simulink model "mrefrobotarm_modified_previous_y_previous_u_previous_ref_pert_2"  (R2018b)
settings: Solver=FixedStepAuto  StartTime=0.0  StopTime=60  RelTol=1e-3  AbsTol=1e-6
undefined symbols (not defined in the file or in its folder): cc, options
libraries: neural x858, simulink x1
(part 30 of 32)

== system mrefrobotarm_modified_previous_y_previous_u_previous_ref_pert_2/m=0.01 sd=0.001/Layer 3/Delays 1 ==
  "p{3}" : Inport  PortDimensions=30
      mask Display: e = 0.06;c1 = [120 230 180]/255;c2 = ([120 230 180]+0)/(256+128);c3 = ([120 230 180]+128)/(256+128);patch([0 1 1 0],[0 0 1 1],c1);patch([0 1 1 1-e 1-e 0+e],[0 0 1 1-e 0+e 0+e],c2);patch([0 0 1 1-e 0+e 0+e],[0 1 1 1-e 1-e 0+e],c3);plot([0 1 1 0 0],[0 0 1 1 0]);
  mux : Mux  Inputs=1
      mask Display: e = 0.06;c1 = [120 150 230]/255;c2 = ([120 150 230]+0)/383;c3 = ([120 150 230]+128)/383;patch([0 1 1 0],[0 0 1 1],c1);patch([0 1 1 1-e 1-e 0+e],[0 0 1 1-e 0+e 0+e],c2);patch([0 0 1 1-e 0+e 0+e],[0 1 1 1-e 1-e 0+e],c3);plot([0 1 1 0 0],[0 0 1 1 0]);disp('Mux')
  "pd{3,2}" : Outport
      mask Display: e = 0.06;c1 = [120 230 180]/255;c2 = ([120 230 180]+0)/(256+128);c3 = ([120 230 180]+128)/(256+128);patch([0 1 1 0],[0 0 1 1],c1);patch([0 1 1 1-e 1-e 0+e],[0 0 1 1-e 0+e 0+e],c2);patch([0 0 1 1-e 0+e 0+e],[0 1 1 1-e 1-e 0+e],c3);plot([0 1 1 0 0],[0 0 1 1 0]);
  wires:
  "p{3}"/1 -> mux/1
  mux/1 -> "pd{3,2}"/1

== system mrefrobotarm_modified_previous_y_previous_u_previous_ref_pert_2/m=0.01 sd=0.001/Layer 3/LW{3,2} ==
  "ad{3,2}" : Inport  PortDimensions=30
      mask Display: e = 0.06;c1 = [120 230 180]/255;c2 = ([120 230 180]+0)/(256+128);c3 = ([120 230 180]+128)/(256+128);patch([0 1 1 0],[0 0 1 1],c1);patch([0 1 1 1-e 1-e 0+e],[0 0 1 1-e 0+e 0+e],c2);patch([0 0 1 1-e 0+e 0+e],[0 1 1 1-e 1-e 0+e],c3);plot([0 1 1 0 0],[0 0 1 1 0]);
  "IW{3,2}(1,:)'" : Constant  Value=[0.243283358953629402776641654781997203826904296875;0.0052243178148873060939738621755168423987925052642822265625;0.0264492508062884081054821905354401678778231143951416015625;0.2454647413544485401448724815054447390139102935791015625;-0.30345238295906995507067449580063112080097198486328125;-0.08772749743109610476299309311798424459993839263916015625;-0.300484076073690486996525805807323195040225982666015625;-0.25574179039630273724270637103472836315631866455078125;-0.4022085380966633483268424242851324379444122314453125;-0.32038735324012412863936560825095511972904205322265625;0.39682017437081473776316897783544845879077911376953125;-0.19002415108010850541830905058304779231548309326171875;0.1034079154633195385404320632005692459642887115478515625;-0.49654610538757726345693299663253128528594970703125;-0.252709011184159615392985642756684683263301849365234375;0.051813445988101620998111940252783824689686298370361328125;-0.119411317170181663360750690117129124701023101806640625;-0.238083190801845312467577286952291615307331085205078125;0.0603028351061200285077035232461639679968357086181640625;0.334975652187224304245916073341504670679569244384765625;-0.40385752692782972417262499220669269561767578125;0.26298542443057371098547037036041729152202606201171875;-0.379084529953288396075805621876497752964496612548828125;-0.330978605194054809057746524558751843869686126708984375;-0.289042778322861571016488824170664884150028228759765625;0.253230096744817612108846560659003444015979766845703125;-0.155565791924000607071576496309717185795307159423828125;0.159285938319768283211175230462686158716678619384765625;-0.28458279469647440595991838563350029289722442626953125;-0.6006058809980039381315464197541587054729461669921875]
      mask Display: e = 0.06;c1 = [120 150 230]/255;c2 = ([120 150 230]+0)/383;c3 = ([120 150 230]+128)/383;patch([0 1 1 0],[0 0 1 1],c1);patch([0 1 1 1-e 1-e 0+e],[0 0 1 1-e 0+e 0+e],c2);patch([0 0 1 1-e 0+e 0+e],[0 1 1 1-e 1-e 0+e],c3);plot([0 1 1 0 0],[0 0 1 1 0]);disp('weights');
  Mux : Mux  Inputs=1
      mask Display: e = 0.06;c1 = [120 150 230]/255;c2 = ([120 150 230]+0)/383;c3 = ([120 150 230]+128)/383;patch([0 1 1 0],[0 0 1 1],c1);patch([0 1 1 1-e 1-e 0+e],[0 0 1 1-e 0+e 0+e],c2);patch([0 0 1 1-e 0+e 0+e],[0 1 1 1-e 1-e 0+e],c3);plot([0 1 1 0 0],[0 0 1 1 0]);disp('Mux');
  dotprod1 : neural/Weight Functions/dotprod
  "lz{3,2}" : Outport
      mask Display: e = 0.06;c1 = [120 230 180]/255;c2 = ([120 230 180]+0)/(256+128);c3 = ([120 230 180]+128)/(256+128);patch([0 1 1 0],[0 0 1 1],c1);patch([0 1 1 1-e 1-e 0+e],[0 0 1 1-e 0+e 0+e],c2);patch([0 0 1 1-e 0+e 0+e],[0 1 1 1-e 1-e 0+e],c3);plot([0 1 1 0 0],[0 0 1 1 0]);
  wires:
  "IW{3,2}(1,:)'"/1 -> dotprod1/1
  "ad{3,2}"/1 -> dotprod1/2
  dotprod1/1 -> Mux/1
  Mux/1 -> "lz{3,2}"/1

== system mrefrobotarm_modified_previous_y_previous_u_previous_ref_pert_2/m=0.1 sd=0.001/Layer 1/Delays 1 ==
  "p{1}" : Inport  PortDimensions=10
      mask Display: e = 0.06;c1 = [120 230 180]/255;c2 = ([120 230 180]+0)/(256+128);c3 = ([120 230 180]+128)/(256+128);patch([0 1 1 0],[0 0 1 1],c1);patch([0 1 1 1-e 1-e 0+e],[0 0 1 1-e 0+e 0+e],c2);patch([0 0 1 1-e 0+e 0+e],[0 1 1 1-e 1-e 0+e],c3);plot([0 1 1 0 0],[0 0 1 1 0]);
  mux : Mux  Inputs=1
      mask Display: e = 0.06;c1 = [120 150 230]/255;c2 = ([120 150 230]+0)/383;c3 = ([120 150 230]+128)/383;patch([0 1 1 0],[0 0 1 1],c1);patch([0 1 1 1-e 1-e 0+e],[0 0 1 1-e 0+e 0+e],c2);patch([0 0 1 1-e 0+e 0+e],[0 1 1 1-e 1-e 0+e],c3);plot([0 1 1 0 0],[0 0 1 1 0]);disp('Mux')
  "pd{1,1}" : Outport
      mask Display: e = 0.06;c1 = [120 230 180]/255;c2 = ([120 230 180]+0)/(256+128);c3 = ([120 230 180]+128)/(256+128);patch([0 1 1 0],[0 0 1 1],c1);patch([0 1 1 1-e 1-e 0+e],[0 0 1 1-e 0+e 0+e],c2);patch([0 0 1 1-e 0+e 0+e],[0 1 1 1-e 1-e 0+e],c3);plot([0 1 1 0 0],[0 0 1 1 0]);
  wires:
  "p{1}"/1 -> mux/1
  mux/1 -> "pd{1,1}"/1

== system mrefrobotarm_modified_previous_y_previous_u_previous_ref_pert_2/m=0.1 sd=0.001/Layer 1/IW{1,1} ==
  "pd{1,1}" : Inport  PortDimensions=10
      mask Display: e = 0.06;c1 = [120 230 180]/255;c2 = ([120 230 180]+0)/(256+128);c3 = ([120 230 180]+128)/(256+128);patch([0 1 1 0],[0 0 1 1],c1);patch([0 1 1 1-e 1-e 0+e],[0 0 1 1-e 0+e 0+e],c2);patch([0 0 1 1-e 0+e 0+e],[0 1 1 1-e 1-e 0+e],c3);plot([0 1 1 0 0],[0 0 1 1 0]);
  "IW{1,1}(1,:)'" : Constant  Value=[0.97150289702667269597924359914031811058521270751953125;0.617885535943719421680953018949367105960845947265625;0.1752264140459464381027743229424231685698032379150390625;-0.0470176874894272234239878116568434052169322967529296875;0.75753700203231832954742230867850594222545623779296875;-0.6427595381168291766016409383155405521392822265625;0.53012825773271554652410486596636474132537841796875;0.6688038187694134162342152194469235837459564208984375;-1.51573934873066917816686327569186687469482421875;-1.8233994053194997331246440808172337710857391357421875]
      mask Display: e = 0.06;c1 = [120 150 230]/255;c2 = ([120 150 230]+0)/383;c3 = ([120 150 230]+128)/383;patch([0 1 1 0],[0 0 1 1],c1);patch([0 1 1 1-e 1-e 0+e],[0 0 1 1-e 0+e 0+e],c2);patch([0 0 1 1-e 0+e 0+e],[0 1 1 1-e 1-e 0+e],c3);plot([0 1 1 0 0],[0 0 1 1 0]);disp('Weights');
  "IW{1,1}(10,:)'" : Constant  Value=[0.489643008794402867511763588481699116528034210205078125;0.249588248674551038686075798977981321513652801513671875;0.4146828443458738799876073244377039372920989990234375;-0.44031407922737153537440235595568083226680755615234375;0.353625460658760715215720438209245912730693817138671875;0.926682652630255621062360660289414227008819580078125;-1.382443840359943720841329195536673069000244140625;-0.280540021092768598887090547577827237546443939208984375;2.600590207035732515095105554792098701000213623046875;0.87696388944716263669221234522410668432712554931640625]
      mask Display: e = 0.06;c1 = [120 150 230]/255;c2 = ([120 150 230]+0)/383;c3 = ([120 150 230]+128)/383;patch([0 1 1 0],[0 0 1 1],c1);patch([0 1 1 1-e 1-e 0+e],[0 0 1 1-e 0+e 0+e],c2);patch([0 0 1 1-e 0+e 0+e],[0 1 1 1-e 1-e 0+e],c3);plot([0 1 1 0 0],[0 0 1 1 0]);disp('Weights');
  "IW{1,1}(11,:)'" : Constant  Value=[-0.4287325006343249977902587488642893731594085693359375;0.2177436358527625459569065924370079301297664642333984375;0.0194862340827772033413634034104688907973468303680419921875;0.384060270608029774574987413870985619723796844482421875;0.8253590670554189490104590731789357960224151611328125;-2.082055111283486414919252638355828821659088134765625;1.23818472207362884063286401215009391307830810546875;0.2379638156625711598035621818780782632529735565185546875;-1.222522228966350876788737878086976706981658935546875;-0.06619512355622218791051381003853748552501201629638671875]
      mask Display: e = 0.06;c1 = [120 150 230]/255;c2 = ([120 150 230]+0)/383;c3 = ([120 150 230]+128)/383;patch([0 1 1 0],[0 0 1 1],c1);patch([0 1 1 1-e 1-e 0+e],[0 0 1 1-e 0+e 0+e],c2);patch([0 0 1 1-e 0+e 0+e],[0 1 1 1-e 1-e 0+e],c3);plot([0 1 1 0 0],[0 0 1 1 0]);disp('Weights');
  "IW{1,1}(12,:)'" : Constant  Value=[-1.2529262660683941899009141707210801541805267333984375;0.2109962353451392547132314803093322552740573883056640625;-0.07807793152172838591074111036505200900137424468994140625;0.06666872948784439978364702028557076118886470794677734375;1.981120844897162669440149329602718353271484375;-2.146903429308871569247685329173691570758819580078125;-0.26792451404853123708704742966801859438419342041015625;0.1142981625892685315637464782412280328571796417236328125;0.4915680538073254890463203992112539708614349365234375;1.042045568544349265494020073674619197845458984375]
      mask Display: e = 0.06;c1 = [120 150 230]/255;c2 = ([120 150 230]+0)/383;c3 = ([120 150 230]+128)/383;patch([0 1 1 0],[0 0 1 1],c1);patch([0 1 1 1-e 1-e 0+e],[0 0 1 1-e 0+e 0+e],c2);patch([0 0 1 1-e 0+e 0+e],[0 1 1 1-e 1-e 0+e],c3);plot([0 1 1 0 0],[0 0 1 1 0]);disp('Weights');
  "IW{1,1}(13,:)'" : Constant  Value=[-1.4694188756818398200465480840648524463176727294921875;0.6336793886650562424023291896446608006954193115234375;2.01225819370897429649858167977072298526763916015625;-0.050672278846553175934985802086885087192058563232421875;-3.23486632336392521125389976077713072299957275390625;2.224412737952894847381912768469192087650299072265625;2.065804235025697987992998605477623641490936279296875;-0.1310957483963151037897887363214977085590362548828125;-0.9522457855727191056161018423154018819332122802734375;-0.1780689484287442947429980222295853309333324432373046875]
      mask Display: e = 0.06;c1 = [120 150 230]/255;c2 = ([120 150 230]+0)/383;c3 = ([120 150 230]+128)/383;patch([0 1 1 0],[0 0 1 1],c1);patch([0 1 1 1-e 1-e 0+e],[0 0 1 1-e 0+e 0+e],c2);patch([0 0 1 1-e 0+e 0+e],[0 1 1 1-e 1-e 0+e],c3);plot([0 1 1 0 0],[0 0 1 1 0]);disp('Weights');
  "IW{1,1}(14,:)'" : Constant  Value=[1.8681607584848112235675898773479275405406951904296875;-1.5591874304554658170474112921510823071002960205078125;0.42450993697366146140126375030376948416233062744140625;-0.1220891736443905362108353074290789663791656494140625;0.763373075356110764033701343578286468982696533203125;-0.2270206585839918134173132102660019882023334503173828125;0.394047816935292838369520040942006744444370269775390625;0.64566378395872436879443512225407175719738006591796875;-0.22964258051511354796758723750826902687549591064453125;0.0630050111280484326226059010878088884055614471435546875]
      mask Display: e = 0.06;c1 = [120 150 230]/255;c2 = ([120 150 230]+0)/383;c3 = ([120 150 230]+128)/383;patch([0 1 1 0],[0 0 1 1],c1);patch([0 1 1 1-e 1-e 0+e],[0 0 1 1-e 0+e 0+e],c2);patch([0 0 1 1-e 0+e 0+e],[0 1 1 1-e 1-e 0+e],c3);plot([0 1 1 0 0],[0 0 1 1 0]);disp('Weights');
  "IW{1,1}(15,:)'" : Constant  Value=[-0.638387118902711048207265775999985635280609130859375;0.93259969282063870377186276527936570346355438232421875;-0.263201104520440820611071330858976580202579498291015625;-0.004599030717388432991377111846986736054532229900360107421875;1.472942132684331273395628159050829708576202392578125;-1.7999757214139944228037393259000964462757110595703125;0.66490212963451345018484062165953218936920166015625;-0.38142345551628842326152835084940306842327117919921875;-0.406565578149011452868677451988332904875278472900390625;-1.131003307321973405663584344438277184963226318359375]
      mask Display: e = 0.06;c1 = [120 150 230]/255;c2 = ([120 150 230]+0)/383;c3 = ([120 150 230]+128)/383;patch([0 1 1 0],[0 0 1 1],c1);patch([0 1 1 1-e 1-e 0+e],[0 0 1 1-e 0+e 0+e],c2);patch([0 0 1 1-e 0+e 0+e],[0 1 1 1-e 1-e 0+e],c3);plot([0 1 1 0 0],[0 0 1 1 0]);disp('Weights');
  "IW{1,1}(16,:)'" : Constant  Value=[-0.43428661364521559118401228261063806712627410888671875;1.007980197023808255352150808903388679027557373046875;-1.1368150682438351584124802684527821838855743408203125;0.046007823780444483119378418223277549259364604949951171875;0.369116877955644240305588255068869329988956451416015625;0.49535162439032187631227088786545209586620330810546875;-0.65503047820462800832075345169869251549243927001953125;0.84142974346925425432885958798578940331935882568359375;0.1335618919760182266021075747630675323307514190673828125;0.200164880680326950912473193966434337198734283447265625]
      mask Display: e = 0.06;c1 = [120 150 230]/255;c2 = ([120 150 230]+0)/383;c3 = ([120 150 230]+128)/383;patch([0 1 1 0],[0 0 1 1],c1);patch([0 1 1 1-e 1-e 0+e],[0 0 1 1-e 0+e 0+e],c2);patch([0 0 1 1-e 0+e 0+e],[0 1 1 1-e 1-e 0+e],c3);plot([0 1 1 0 0],[0 0 1 1 0]);disp('Weights');
  "IW{1,1}(17,:)'" : Constant  Value=[0.107552759922356966360013075245660729706287384033203125;-1.346270777388516304284848956740461289882659912109375;0.184320209842593396576404529696446843445301055908203125;-0.0895953581737940485396620715619064867496490478515625;0.981520970911235135503147830604575574398040771484375;1.02736081963616943113493107375688850879669189453125;-1.1863162004389049553054746866109780967235565185546875;0.283045855992447581428450575913302600383758544921875;-1.392742600295459709514034329913556575775146484375;0.1495563049644798858661687290805275551974773406982421875]
      mask Display: e = 0.06;c1 = [120 150 230]/255;c2 = ([120 150 230]+0)/383;c3 = ([120 150 230]+128)/383;patch([0 1 1 0],[0 0 1 1],c1);patch([0 1 1 1-e 1-e 0+e],[0 0 1 1-e 0+e 0+e],c2);patch([0 0 1 1-e 0+e 0+e],[0 1 1 1-e 1-e 0+e],c3);plot([0 1 1 0 0],[0 0 1 1 0]);disp('Weights');
  "IW{1,1}(18,:)'" : Constant  Value=[0.60421323192831499770960590467439033091068267822265625;0.863981081042938026115507454960606992244720458984375;-2.164800667863084893127734176232479512691497802734375;-0.07698153501303210688444522702411632053554058074951171875;-2.2141952501059449787135235965251922607421875;0.48418268786651286195166221659746952354907989501953125;0.1804086706541263851466538881140877492725849151611328125;-0.483357613735531099763420570525340735912322998046875;-2.250245781538189770998314997996203601360321044921875;-1.889499368656487376938457600772380828857421875]
      mask Display: e = 0.06;c1 = [120 150 230]/255;c2 = ([120 150 230]+0)/383;c3 = ([120 150 230]+128)/383;patch([0 1 1 0],[0 0 1 1],c1);patch([0 1 1 1-e 1-e 0+e],[0 0 1 1-e 0+e 0+e],c2);patch([0 0 1 1-e 0+e 0+e],[0 1 1 1-e 1-e 0+e],c3);plot([0 1 1 0 0],[0 0 1 1 0]);disp('Weights');
  "IW{1,1}(19,:)'" : Constant  Value=[-0.310316878774572646459972702359664253890514373779296875;-1.0780002166131661400783059434616006910800933837890625;0.97905383674770185553626333785359747707843780517578125;0.25263709689869118246718926457106135785579681396484375;0.198392588265190017438044378650374710559844970703125;1.958092704212322399115464577334932982921600341796875;-0.57605587336904939821380366993253119289875030517578125;-1.2966037305212319008518306873156689107418060302734375;1.1480352853282782543686835197149775922298431396484375;0.48066285180312073865849242793046869337558746337890625]
      mask Display: e = 0.06;c1 = [120 150 230]/255;c2 = ([120 150 230]+0)/383;c3 = ([120 150 230]+128)/383;patch([0 1 1 0],[0 0 1 1],c1);patch([0 1 1 1-e 1-e 0+e],[0 0 1 1-e 0+e 0+e],c2);patch([0 0 1 1-e 0+e 0+e],[0 1 1 1-e 1-e 0+e],c3);plot([0 1 1 0 0],[0 0 1 1 0]);disp('Weights');
  "IW{1,1}(2,:)'" : Constant  Value=[0.3387257184963281542167123916442506015300750732421875;-0.1797003643190983879218691754431347362697124481201171875;0.356085463904586119188167003812850452959537506103515625;-0.042189007117119099732338582953161676414310932159423828125;-1.649270794860369537815358853549696505069732666015625;1.464964797139139296433540948783047497272491455078125;-0.7069449258673403679864577497937716543674468994140625;0.61437488507698201356532763384166173636913299560546875;-0.2265416857285133256372233745423727668821811676025390625;0.376347036314308047710852633827016688883304595947265625]
      mask Display: e = 0.06;c1 = [120 150 230]/255;c2 = ([120 150 230]+0)/383;c3 = ([120 150 230]+128)/383;patch([0 1 1 0],[0 0 1 1],c1);patch([0 1 1 1-e 1-e 0+e],[0 0 1 1-e 0+e 0+e],c2);patch([0 0 1 1-e 0+e 0+e],[0 1 1 1-e 1-e 0+e],c3);plot([0 1 1 0 0],[0 0 1 1 0]);disp('Weights');
  "IW{1,1}(20,:)'" : Constant  Value=[-0.490140303142504396571865754594909958541393280029296875;0.79804833937093355711311915001715533435344696044921875;-1.2831688138474799387722669052891433238983154296875;0.291284969844939178873488572207861579954624176025390625;0.876417228536505721336880014860071241855621337890625;-1.7385563549437661468033411438227631151676177978515625;-0.50686148598950564458931467015645466744899749755859375;-0.28939862193536092238588253167108632624149322509765625;-1.2296078733237567615077523441868834197521209716796875;-1.57640760470990759500864442088641226291656494140625]
      mask Display: e = 0.06;c1 = [120 150 230]/255;c2 = ([120 150 230]+0)/383;c3 = ([120 150 230]+128)/383;patch([0 1 1 0],[0 0 1 1],c1);patch([0 1 1 1-e 1-e 0+e],[0 0 1 1-e 0+e 0+e],c2);patch([0 0 1 1-e 0+e 0+e],[0 1 1 1-e 1-e 0+e],c3);plot([0 1 1 0 0],[0 0 1 1 0]);disp('Weights');
  "IW{1,1}(21,:)'" : Constant  Value=[-0.8448419884512754496341813137405551970005035400390625;0.110704272323804142619252388612949289381504058837890625;0.6221730601826127582398839876987040042877197265625;-0.0094678207165062276684519559921682230196893215179443359375;-1.008898321112665197318847276619635522365570068359375;2.37691406571895935684324285830371081829071044921875;-0.98396704720915695308036674759932793676853179931640625;-0.301532716218349261527720273079467006027698516845703125;0.401508735767118707382650200088392011821269989013671875;0.48074242408417700023193219749373383820056915283203125]
      mask Display: e = 0.06;c1 = [120 150 230]/255;c2 = ([120 150 230]+0)/383;c3 = ([120 150 230]+128)/383;patch([0 1 1 0],[0 0 1 1],c1);patch([0 1 1 1-e 1-e 0+e],[0 0 1 1-e 0+e 0+e],c2);patch([0 0 1 1-e 0+e 0+e],[0 1 1 1-e 1-e 0+e],c3);plot([0 1 1 0 0],[0 0 1 1 0]);disp('Weights');
  "IW{1,1}(22,:)'" : Constant  Value=[-0.54005738902516398081132820152561180293560028076171875;1.6497089693146007594037882881821133196353912353515625;0.68022190254479852900004743787576444447040557861328125;-0.11952988714669064707063483865567832253873348236083984375;-2.191214874887081887067097341059707105159759521484375;0.823576955060695947707927189185284078121185302734375;2.546953080893350485069959177053533494472503662109375;-0.1184862413534755187782820939901284873485565185546875;-1.80301440869707452208103859447874128818511962890625;-0.5395918499269087842407088828622363507747650146484375]
      mask Display: e = 0.06;c1 = [120 150 230]/255;c2 = ([120 150 230]+0)/383;c3 = ([120 150 230]+128)/383;patch([0 1 1 0],[0 0 1 1],c1);patch([0 1 1 1-e 1-e 0+e],[0 0 1 1-e 0+e 0+e],c2);patch([0 0 1 1-e 0+e 0+e],[0 1 1 1-e 1-e 0+e],c3);plot([0 1 1 0 0],[0 0 1 1 0]);disp('Weights');
  "IW{1,1}(23,:)'" : Constant  Value=[0.1111125952273283867821618287052842788398265838623046875;-0.125837860955586411382256528668222017586231231689453125;-1.0573139259908701514945050803362391889095306396484375;0.0199283896174118069222203075696597807109355926513671875;0.315679639236594311579864324812660925090312957763671875;0.42717506618387834915751000153250060975551605224609375;-0.25276948903202633989195646790903992950916290283203125;0.37217397859028211737353331045596860349178314208984375;-0.047986027660040307674105264368336065672338008880615234375;-0.71436988024424419307933931122533977031707763671875]
      mask Display: e = 0.06;c1 = [120 150 230]/255;c2 = ([120 150 230]+0)/383;c3 = ([120 150 230]+128)/383;patch([0 1 1 0],[0 0 1 1],c1);patch([0 1 1 1-e 1-e 0+e],[0 0 1 1-e 0+e 0+e],c2);patch([0 0 1 1-e 0+e 0+e],[0 1 1 1-e 1-e 0+e],c3);plot([0 1 1 0 0],[0 0 1 1 0]);disp('Weights');
  "IW{1,1}(24,:)'" : Constant  Value=[0.6031876739999459946517390562803484499454498291015625;-1.36680629289936206305355881340801715850830078125;0.439752228564215530415282273679622448980808258056640625;0.313991143349557189079490626681945286691188812255859375;-0.5705459948731419483891613708692602813243865966796875;1.03530481535340346255225085769779980182647705078125;-0.59872468406984113986624151948490180075168609619140625;-0.1399879051014731590196760180333512835204601287841796875;0.190202809094372649045823209235095418989658355712890625;0.0005722435480554452676138499356284228269942104816436767578125]
      mask Display: e = 0.06;c1 = [120 150 230]/255;c2 = ([120 150 230]+0)/383;c3 = ([120 150 230]+128)/383;patch([0 1 1 0],[0 0 1 1],c1);patch([0 1 1 1-e 1-e 0+e],[0 0 1 1-e 0+e 0+e],c2);patch([0 0 1 1-e 0+e 0+e],[0 1 1 1-e 1-e 0+e],c3);plot([0 1 1 0 0],[0 0 1 1 0]);disp('Weights');
  "IW{1,1}(25,:)'" : Constant  Value=[-0.471166329686002638421626897979876957833766937255859375;0.019517284199158567437049072168520069681107997894287109375;-0.51375562108899142099716073062154464423656463623046875;-0.99099158086243332999032418229035101830959320068359375;-0.280529395720106877742949791354476474225521087646484375;0.408813229901232200180771769737475551664829254150390625;-1.4569675807901523167942059444612823426723480224609375;0.1597914239924210499932399898170842789113521575927734375;-1.151683674628356524038963470957241952419281005859375;-1.1155745139129293885815741305123083293437957763671875]
      mask Display: e = 0.06;c1 = [120 150 230]/255;c2 = ([120 150 230]+0)/383;c3 = ([120 150 230]+128)/383;patch([0 1 1 0],[0 0 1 1],c1);patch([0 1 1 1-e 1-e 0+e],[0 0 1 1-e 0+e 0+e],c2);patch([0 0 1 1-e 0+e 0+e],[0 1 1 1-e 1-e 0+e],c3);plot([0 1 1 0 0],[0 0 1 1 0]);disp('Weights');
  "IW{1,1}(26,:)'" : Constant  Value=[0.51788957071500363316118864531745202839374542236328125;-0.90550825047783722876459933104342781007289886474609375;0.874554192761201054651110098347999155521392822265625;0.05490630649626752901593107480948674492537975311279296875;-0.2376871617598398100934531385064474307000637054443359375;-1.4259068300949875318650583722046576440334320068359375;1.56037911854196753580481527023948729038238525390625;-0.5633426023816168193292241994640789926052093505859375;-0.3249990459048144320064466228359378874301910400390625;-0.1924690193035773211338579358198330737650394439697265625]
      mask Display: e = 0.06;c1 = [120 150 230]/255;c2 = ([120 150 230]+0)/383;c3 = ([120 150 230]+128)/383;patch([0 1 1 0],[0 0 1 1],c1);patch([0 1 1 1-e 1-e 0+e],[0 0 1 1-e 0+e 0+e],c2);patch([0 0 1 1-e 0+e 0+e],[0 1 1 1-e 1-e 0+e],c3);plot([0 1 1 0 0],[0 0 1 1 0]);disp('Weights');
  "IW{1,1}(27,:)'" : Constant  Value=[0.4086370536036636469390259662759490311145782470703125;-0.2007808125360639184275868274198728613555431365966796875;0.60343773748294415870674356483505107462406158447265625;1.070394363751332900136503667454235255718231201171875;2.2073601470784325329077546484768390655517578125;0.25483112077533653927474688316578976809978485107421875;-0.33905692912207296974003156719845719635486602783203125;-0.7065582091683511034574394216178916394710540771484375;-0.60042970740870671431110849880496971309185028076171875;-0.1279585049280285991013528246185160242021083831787109375]
      mask Display: e = 0.06;c1 = [120 150 230]/255;c2 = ([120 150 230]+0)/383;c3 = ([120 150 230]+128)/383;patch([0 1 1 0],[0 0 1 1],c1);patch([0 1 1 1-e 1-e 0+e],[0 0 1 1-e 0+e 0+e],c2);patch([0 0 1 1-e 0+e 0+e],[0 1 1 1-e 1-e 0+e],c3);plot([0 1 1 0 0],[0 0 1 1 0]);disp('Weights');
  "IW{1,1}(28,:)'" : Constant  Value=[-0.17889977814008284351388056165887974202632904052734375;-0.72737896249138522808408424680237658321857452392578125;0.876562342050114740032995541696436703205108642578125;0.06250436501011306933417444042788702063262462615966796875;0.98605104672372723140227890326059423387050628662109375;-0.0177154137537540203040098418796333135105669498443603515625;-1.1565789570964295496224849557620473206043243408203125;0.05094103404277350310991323567577637732028961181640625;0.53028155866240200833061635421472601592540740966796875;-0.637525850452747899765881811617873609066009521484375]
      mask Display: e = 0.06;c1 = [120 150 230]/255;c2 = ([120 150 230]+0)/383;c3 = ([120 150 230]+128)/383;patch([0 1 1 0],[0 0 1 1],c1);patch([0 1 1 1-e 1-e 0+e],[0 0 1 1-e 0+e 0+e],c2);patch([0 0 1 1-e 0+e 0+e],[0 1 1 1-e 1-e 0+e],c3);plot([0 1 1 0 0],[0 0 1 1 0]);disp('Weights');
  "IW{1,1}(29,:)'" : Constant  Value=[0.183816634740196216402097206810140050947666168212890625;-0.605890372960407486147005329257808625698089599609375;-0.52787986615784898702941063675098121166229248046875;0.3209207542221850228969515228527598083019256591796875;0.392028568404616972742360303527675569057464599609375;-0.71187172137459153731242622598074376583099365234375;0.1788547241704122325867132303756079636514186859130859375;0.89792898555716738062670856379554606974124908447265625;-0.80277707368138362387099959960323758423328399658203125;0.8280432752455038070138471084646880626678466796875]
      mask Display: e = 0.06;c1 = [120 150 230]/255;c2 = ([120 150 230]+0)/383;c3 = ([120 150 230]+128)/383;patch([0 1 1 0],[0 0 1 1],c1);patch([0 1 1 1-e 1-e 0+e],[0 0 1 1-e 0+e 0+e],c2);patch([0 0 1 1-e 0+e 0+e],[0 1 1 1-e 1-e 0+e],c3);plot([0 1 1 0 0],[0 0 1 1 0]);disp('Weights');
  "IW{1,1}(3,:)'" : Constant  Value=[-0.62632140158312987754385403604828752577304840087890625;-0.52645332897737973087970431151916272938251495361328125;0.422629068709391930713792362439562566578388214111328125;0.16303550788070542143515240240958519279956817626953125;1.162694599040965837133398963487707078456878662109375;-0.1394240777189013069659040411352179944515228271484375;0.02236044267614045732983640846214257180690765380859375;0.309760520161516395010181668112636543810367584228515625;-1.2335632156852314178507867836742661893367767333984375;-0.66691887772808045031780466160853393375873565673828125]
      mask Display: e = 0.06;c1 = [120 150 230]/255;c2 = ([120 150 230]+0)/383;c3 = ([120 150 230]+128)/383;patch([0 1 1 0],[0 0 1 1],c1);patch([0 1 1 1-e 1-e 0+e],[0 0 1 1-e 0+e 0+e],c2);patch([0 0 1 1-e 0+e 0+e],[0 1 1 1-e 1-e 0+e],c3);plot([0 1 1 0 0],[0 0 1 1 0]);disp('Weights');
  "IW{1,1}(30,:)'" : Constant  Value=[-1.0466886010133702455959792132489383220672607421875;1.0555506401177241482258750693290494382381439208984375;-0.370726708404341021019234858613344840705394744873046875;0.068745345313962591404788327054120600223541259765625;-0.462596703918887020012817856695619411766529083251953125;-0.58865942656746172989556953325518406927585601806640625;0.7620448134768500469959917609230615198612213134765625;-0.09112676064769120731767770848819054663181304931640625;0.174174231500589804522149961485411040484905242919921875;-0.44108843496463323585743410149007104337215423583984375]
      mask Display: e = 0.06;c1 = [120 150 230]/255;c2 = ([120 150 230]+0)/383;c3 = ([120 150 230]+128)/383;patch([0 1 1 0],[0 0 1 1],c1);patch([0 1 1 1-e 1-e 0+e],[0 0 1 1-e 0+e 0+e],c2);patch([0 0 1 1-e 0+e 0+e],[0 1 1 1-e 1-e 0+e],c3);plot([0 1 1 0 0],[0 0 1 1 0]);disp('Weights');
  "IW{1,1}(4,:)'" : Constant  Value=[0.42184809618783625229099243370001204311847686767578125;0.57438939445128822658404033063561655580997467041015625;0.139608219524607779504776772228069603443145751953125;-0.0607540974594706906231067478074692189693450927734375;1.38227605926035579386734752915799617767333984375;-1.602370341086080340886610429151915013790130615234375;-0.342482978911408053601661549691925756633281707763671875;0.80767878669071635489018490261514671146869659423828125;0.79082152886633405586280787247233092784881591796875;-0.7645203885690905476479883873253129422664642333984375]
      mask Display: e = 0.06;c1 = [120 150 230]/255;c2 = ([120 150 230]+0)/383;c3 = ([120 150 230]+128)/383;patch([0 1 1 0],[0 0 1 1],c1);patch([0 1 1 1-e 1-e 0+e],[0 0 1 1-e 0+e 0+e],c2);patch([0 0 1 1-e 0+e 0+e],[0 1 1 1-e 1-e 0+e],c3);plot([0 1 1 0 0],[0 0 1 1 0]);disp('Weights');
  "IW{1,1}(5,:)'" : Constant  Value=[0.60691098084142769408799722441472113132476806640625;0.08894199181516516949930206692442880012094974517822265625;-0.00837926756515577735029420836099234293214976787567138671875;0.0696532879566251483804961708301561884582042694091796875;0.483676615247791874541150036748149432241916656494140625;0.332173416716467773124321638533729128539562225341796875;-1.0188183642328054734349507270962931215763092041015625;0.46527057400741533843557817817782051861286163330078125;0.9512447102577112900689826346933841705322265625;-0.84098851707301403024530372931621968746185302734375]
      mask Display: e = 0.06;c1 = [120 150 230]/255;c2 = ([120 150 230]+0)/383;c3 = ([120 150 230]+128)/383;patch([0 1 1 0],[0 0 1 1],c1);patch([0 1 1 1-e 1-e 0+e],[0 0 1 1-e 0+e 0+e],c2);patch([0 0 1 1-e 0+e 0+e],[0 1 1 1-e 1-e 0+e],c3);plot([0 1 1 0 0],[0 0 1 1 0]);disp('Weights');
  "IW{1,1}(6,:)'" : Constant  Value=[1.4712226032100961248261228320188820362091064453125;-0.356180687758446357094044287805445492267608642578125;0.11390358287453027086311152515918365679681301116943359375;-0.0348426358868414165481652844391646794974803924560546875;3.822214954005693332561577335582114756107330322265625;-0.80816876436139273298664420508430339395999908447265625;-1.7619207714984821411263737900299020111560821533203125;-0.340113332533821421943542873123078607022762298583984375;-0.0644091818982337194210430197927053086459636688232421875;0.3464644391002706935722699199686758220195770263671875]
      mask Display: e = 0.06;c1 = [120 150 230]/255;c2 = ([120 150 230]+0)/383;c3 = ([120 150 230]+128)/383;patch([0 1 1 0],[0 0 1 1],c1);patch([0 1 1 1-e 1-e 0+e],[0 0 1 1-e 0+e 0+e],c2);patch([0 0 1 1-e 0+e 0+e],[0 1 1 1-e 1-e 0+e],c3);plot([0 1 1 0 0],[0 0 1 1 0]);disp('Weights');
  "IW{1,1}(7,:)'" : Constant  Value=[0.07993039207707407223235662740989937447011470794677734375;1.3131166877254549785192239141906611621379852294921875;-1.1123302079079320225929450316471047699451446533203125;-0.52757831174058955614469823558465577661991119384765625;1.0961388390581217056052309999358840286731719970703125;0.8087051288913962299176318992977030575275421142578125;0.5784665545795879548762741251266561448574066162109375;0.0031180074670162532569916979952040492207743227481842041015625;0.20838352352040201420635412432602606713771820068359375;1.33005789594791767882497879327274858951568603515625]
      mask Display: e = 0.06;c1 = [120 150 230]/255;c2 = ([120 150 230]+0)/383;c3 = ([120 150 230]+128)/383;patch([0 1 1 0],[0 0 1 1],c1);patch([0 1 1 1-e 1-e 0+e],[0 0 1 1-e 0+e 0+e],c2);patch([0 0 1 1-e 0+e 0+e],[0 1 1 1-e 1-e 0+e],c3);plot([0 1 1 0 0],[0 0 1 1 0]);disp('Weights');
  "IW{1,1}(8,:)'" : Constant  Value=[-1.6428707822842678609731592587195336818695068359375;0.7770685144406497268931843791506253182888031005859375;0.337837851581247239352023825631476938724517822265625;0.40649067634497992873576777128619141876697540283203125;-0.99206893422060715703736377690802328288555145263671875;0.349530934351896360734457402941188775002956390380859375;0.1060028173692990904886102043747087009251117706298828125;-0.109228967052619807542868102245847694575786590576171875;0.51763383250094907594984761090017855167388916015625;0.98950818573566101665761607364402152597904205322265625]
      mask Display: e = 0.06;c1 = [120 150 230]/255;c2 = ([120 150 230]+0)/383;c3 = ([120 150 230]+128)/383;patch([0 1 1 0],[0 0 1 1],c1);patch([0 1 1 1-e 1-e 0+e],[0 0 1 1-e 0+e 0+e],c2);patch([0 0 1 1-e 0+e 0+e],[0 1 1 1-e 1-e 0+e],c3);plot([0 1 1 0 0],[0 0 1 1 0]);disp('Weights');
  "IW{1,1}(9,:)'" : Constant  Value=[-0.55756270167286914318793833444942720234394073486328125;0.5477373003993297739810941493487916886806488037109375;0.40970147464440664908380540509824641048908233642578125;-0.28692440500681171133834368447423912584781646728515625;1.360631966197447528799102656194008886814117431640625;-2.159319734604072227313054099795408546924591064453125;0.77909457698656847668416958185844123363494873046875;-0.118633661182634686515058319855597801506519317626953125;0.289991601202789384128521987804560922086238861083984375;-0.1904343717402545987926743009666097350418567657470703125]
      mask Display: e = 0.06;c1 = [120 150 230]/255;c2 = ([120 150 230]+0)/383;c3 = ([120 150 230]+128)/383;patch([0 1 1 0],[0 0 1 1],c1);patch([0 1 1 1-e 1-e 0+e],[0 0 1 1-e 0+e 0+e],c2);patch([0 0 1 1-e 0+e 0+e],[0 1 1 1-e 1-e 0+e],c3);plot([0 1 1 0 0],[0 0 1 1 0]);disp('Weights');
  Mux : Mux  Inputs=30
      mask Display: e = 0.06;c1 = [120 150 230]/255;c2 = ([120 150 230]+0)/383;c3 = ([120 150 230]+128)/383;patch([0 1 1 0],[0 0 1 1],c1);patch([0 1 1 1-e 1-e 0+e],[0 0 1 1-e 0+e 0+e],c2);patch([0 0 1 1-e 0+e 0+e],[0 1 1 1-e 1-e 0+e],c3);plot([0 1 1 0 0],[0 0 1 1 0]);disp('Mux');
  dotprod{1..30} (30 alike) : neural/Weight Functions/dotprod
  "iz{1,1}" : Outport
      mask Display: e = 0.06;c1 = [120 230 180]/255;c2 = ([120 230 180]+0)/(256+128);c3 = ([120 230 180]+128)/(256+128);patch([0 1 1 0],[0 0 1 1],c1);patch([0 1 1 1-e 1-e 0+e],[0 0 1 1-e 0+e 0+e],c2);patch([0 0 1 1-e 0+e 0+e],[0 1 1 1-e 1-e 0+e],c3);plot([0 1 1 0 0],[0 0 1 1 0]);
  wires:
  "IW{1,1}(1,:)'"/1 -> dotprod1/1
  "pd{1,1}"/1 -> dotprod1/2, dotprod2/2, dotprod3/2, dotprod4/2, dotprod5/2, dotprod6/2, dotprod7/2, dotprod8/2, dotprod9/2, dotprod10/2, dotprod11/2, dotprod12/2, dotprod13/2, dotprod14/2, dotprod15/2, dotprod16/2, dotprod17/2, dotprod18/2, dotprod19/2, dotprod20/2, dotprod21/2, dotprod22/2, dotprod23/2, dotprod24/2, dotprod25/2, dotprod26/2, dotprod27/2, dotprod28/2, dotprod29/2, dotprod30/2
  dotprod1/1 -> Mux/1
  "IW{1,1}(2,:)'"/1 -> dotprod2/1
  dotprod2/1 -> Mux/2
  "IW{1,1}(3,:)'"/1 -> dotprod3/1
  dotprod3/1 -> Mux/3
  "IW{1,1}(4,:)'"/1 -> dotprod4/1
  dotprod4/1 -> Mux/4
  "IW{1,1}(5,:)'"/1 -> dotprod5/1
  dotprod5/1 -> Mux/5
  "IW{1,1}(6,:)'"/1 -> dotprod6/1
  dotprod6/1 -> Mux/6
  "IW{1,1}(7,:)'"/1 -> dotprod7/1
  dotprod7/1 -> Mux/7
  "IW{1,1}(8,:)'"/1 -> dotprod8/1
  dotprod8/1 -> Mux/8
  "IW{1,1}(9,:)'"/1 -> dotprod9/1
  dotprod9/1 -> Mux/9
  "IW{1,1}(10,:)'"/1 -> dotprod10/1
  dotprod10/1 -> Mux/10
  "IW{1,1}(11,:)'"/1 -> dotprod11/1
  dotprod11/1 -> Mux/11
  "IW{1,1}(12,:)'"/1 -> dotprod12/1
  dotprod12/1 -> Mux/12
  "IW{1,1}(13,:)'"/1 -> dotprod13/1
  dotprod13/1 -> Mux/13
  "IW{1,1}(14,:)'"/1 -> dotprod14/1
  dotprod14/1 -> Mux/14
  "IW{1,1}(15,:)'"/1 -> dotprod15/1
  dotprod15/1 -> Mux/15
  "IW{1,1}(16,:)'"/1 -> dotprod16/1
  dotprod16/1 -> Mux/16
  "IW{1,1}(17,:)'"/1 -> dotprod17/1
  dotprod17/1 -> Mux/17
  "IW{1,1}(18,:)'"/1 -> dotprod18/1
  dotprod18/1 -> Mux/18
  "IW{1,1}(19,:)'"/1 -> dotprod19/1
  dotprod19/1 -> Mux/19
  "IW{1,1}(20,:)'"/1 -> dotprod20/1
  dotprod20/1 -> Mux/20
  "IW{1,1}(21,:)'"/1 -> dotprod21/1
  dotprod21/1 -> Mux/21
  "IW{1,1}(22,:)'"/1 -> dotprod22/1
  dotprod22/1 -> Mux/22
  "IW{1,1}(23,:)'"/1 -> dotprod23/1
  dotprod23/1 -> Mux/23
  "IW{1,1}(24,:)'"/1 -> dotprod24/1
  dotprod24/1 -> Mux/24
  "IW{1,1}(25,:)'"/1 -> dotprod25/1
  dotprod25/1 -> Mux/25
  "IW{1,1}(26,:)'"/1 -> dotprod26/1
  dotprod26/1 -> Mux/26
  "IW{1,1}(27,:)'"/1 -> dotprod27/1
  dotprod27/1 -> Mux/27
  "IW{1,1}(28,:)'"/1 -> dotprod28/1
  dotprod28/1 -> Mux/28
  "IW{1,1}(29,:)'"/1 -> dotprod29/1
  dotprod29/1 -> Mux/29
  "IW{1,1}(30,:)'"/1 -> dotprod30/1
  dotprod30/1 -> Mux/30
  Mux/1 -> "iz{1,1}"/1

== system mrefrobotarm_modified_previous_y_previous_u_previous_ref_pert_2/m=0.1 sd=0.001/Layer 2/Delays 1 ==
  "p{2}" : Inport  PortDimensions=30
      mask Display: e = 0.06;c1 = [120 230 180]/255;c2 = ([120 230 180]+0)/(256+128);c3 = ([120 230 180]+128)/(256+128);patch([0 1 1 0],[0 0 1 1],c1);patch([0 1 1 1-e 1-e 0+e],[0 0 1 1-e 0+e 0+e],c2);patch([0 0 1 1-e 0+e 0+e],[0 1 1 1-e 1-e 0+e],c3);plot([0 1 1 0 0],[0 0 1 1 0]);
  mux : Mux  Inputs=1
      mask Display: e = 0.06;c1 = [120 150 230]/255;c2 = ([120 150 230]+0)/383;c3 = ([120 150 230]+128)/383;patch([0 1 1 0],[0 0 1 1],c1);patch([0 1 1 1-e 1-e 0+e],[0 0 1 1-e 0+e 0+e],c2);patch([0 0 1 1-e 0+e 0+e],[0 1 1 1-e 1-e 0+e],c3);plot([0 1 1 0 0],[0 0 1 1 0]);disp('Mux')
  "pd{2,1}" : Outport
      mask Display: e = 0.06;c1 = [120 230 180]/255;c2 = ([120 230 180]+0)/(256+128);c3 = ([120 230 180]+128)/(256+128);patch([0 1 1 0],[0 0 1 1],c1);patch([0 1 1 1-e 1-e 0+e],[0 0 1 1-e 0+e 0+e],c2);patch([0 0 1 1-e 0+e 0+e],[0 1 1 1-e 1-e 0+e],c3);plot([0 1 1 0 0],[0 0 1 1 0]);
  wires:
  "p{2}"/1 -> mux/1
  mux/1 -> "pd{2,1}"/1
